simulink model "DroneControlSimulink"  (R2023a)
settings: Solver=ode5  StartTime=0.0  StopTime=30  FixedStep=0.01  RelTol=1e-3
values from neighbouring files (symbols this model uses):
  A = eval(A)    [DroneControlm.m]
  A_o = eval(A_o)    [DroneControlm.m]
  B = eval(B)    [DroneControlm.m]
  B_o = eval(B_o)    [DroneControlm.m]
  C = [1 0 0 0 0 0;0 0 1 0 0 0]    [DroneControlm.m]
  C_o = [1 0 0 0 0 0 0 1 ;0 0 1 0 0 0 1 0]    [DroneControlm.m]
  g = 9.81    [DroneControlm.m]
  h = 0.2    [DroneControlm.m]
  I = 0.003    [DroneControlm.m]
  Ic_xl = [0;0;0;0;0;0]    [DroneControlm.m]
  Ic_xnl = Ic_xl+x_nom    [DroneControlm.m]
  K = lqr(Ab,Bb,Q,R)    [DroneControlm.m]
  L = 0.35    [DroneControlm.m]
  L_o = place(A_o',C_o',D_o)'    [DroneControlm.m]
  m = 1.0    (= 1)    [DroneControlm.m]
  u_nom = eval(u_nom)    [DroneControlm.m]
  x_nom = double(x_nom)    [DroneControlm.m]
libraries: vrlib x2, robotcorelib x1
settings Model: Creator=emuca  LastModifiedBy=omert
settings SolverCC: AlgebraicLoopSolver=TrustRegion
settings DebuggingCC: UnconnectedInputMsg=warning  UnconnectedOutputMsg=warning  UnconnectedLineMsg=warning
settings ModelReferenceCC: EnableRefExpFcnMdlSchedulingChecks=on
settings RTWCC: DLArmComputeVersion=19.05

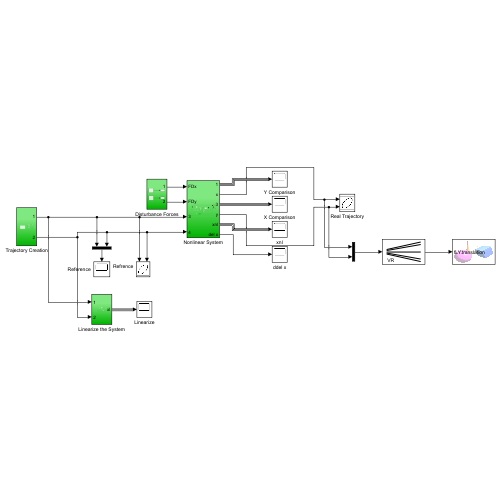
[thumbnail: Simulink's stored preview of the top-level diagram]
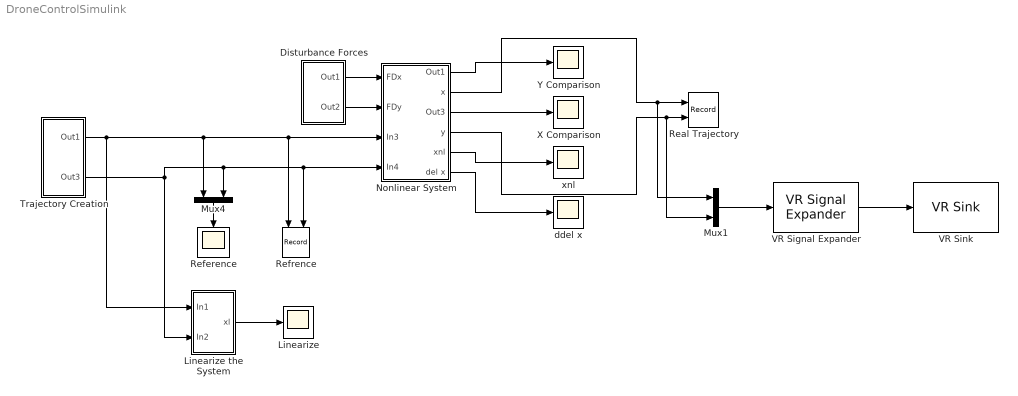
== system DroneControlSimulink ==
  Disturbance Forces : Subsystem
  Linearize : Scope
  Linearize the System : Subsystem
  Mux1 : Mux  Inputs=2
  Mux4 : Mux  Inputs=2
  Nonlinear System : Subsystem
  Real Trajectory : Record  FileSettingsInternal="{\"entries\":[{\"content\":{\"excelSettings\":{\"content\":{},\"type\":\"Streamout.ExcelSettings\"}},\"type\":\"Streamout.FileSettingStorage\",\"uuid\":\"\"}],\"packageUris\":[\"http:\\/\\/schema.mathworks.com\\/mf0\\/streamout_blocks\\/R2020a\"],\"version\":\"1.0\"}"  Layout=[1 1]  SignalsInternal="{\"entries\":[{\"content\":{\"signals\":[{\"content\":{\"blockPath\":[],\"dimensions\":[1],\"domain\":\"\",\"lineColor\":\"#a2142f\",\"plots\":[1],\"port\":1,\"sid\":[\"\"],\"signalID\":4664,\"signalName\":\"Nonlinear System:2\"},\"type\":\"RecordBlkView.Signal\",\"uuid\":\"\"},{\"content\":{\"blockPath\":[],\"dimensions\":[1],\"domain\":\"\",\"lineColor\":\"#139fff\",\"plots\":[1],\"port\":2,\"sid\":[\"\"],\"signalID\":4668,\"signalName\":\"Nonlinear System:4\"},\"type\":\"RecordBlkView.Signal\",\"uuid\":\"\"}]},\"type\":\"RecordBlkView.InputSignals\",\"uuid\":\"\"}],\"packageUris\":[\"http:\\/\\/schema.mathworks.com\\/mf0\\/streamout_blocks\\/R2020a\"],\"version\":\"1.0\"}"  VisualizationBindings="{\"xyplotplugin\":{\"info\":[{\"series\":[{\"bindingParametersList\":[{\"parameter\":\"X-Axis\",\"signalID\":4664,\"signalName\":\"Nonlinear System:2\"},{\"parameter\":\"Y-Axis\",\"signalID\":4668,\"signalName\":\"Nonlinear System:4\"}],\"seriesID\":43140}],\"subplotID\":1}]}}"  CompatibilityTag=XY  st=-1
  Reference : Scope
  "Refrence " : Record  FileSettingsInternal="{\"entries\":[{\"content\":{\"excelSettings\":{\"content\":{},\"type\":\"Streamout.ExcelSettings\"}},\"type\":\"Streamout.FileSettingStorage\",\"uuid\":\"\"}],\"packageUris\":[\"http:\\/\\/schema.mathworks.com\\/mf0\\/streamout_blocks\\/R2020a\"],\"version\":\"1.0\"}"  Layout=[1 1]  SignalsInternal="{\"entries\":[{\"content\":{\"signals\":[{\"content\":{\"blockPath\":[],\"dimensions\":[1],\"domain\":\"\",\"lineColor\":\"#a2142f\",\"plots\":[1],\"port\":1,\"sid\":[\"\"],\"signalID\":4672,\"signalName\":\"Trajectory Creation:1\"},\"type\":\"RecordBlkView.Signal\",\"uuid\":\"\"},{\"content\":{\"blockPath\":[],\"dimensions\":[1],\"domain\":\"\",\"lineColor\":\"#139fff\",\"plots\":[1],\"port\":2,\"sid\":[\"\"],\"signalID\":4676,\"signalName\":\"Trajectory Creation:2\"},\"type\":\"RecordBlkView.Signal\",\"uuid\":\"\"}]},\"type\":\"RecordBlkView.InputSignals\",\"uuid\":\"\"}],\"packageUris\":[\"http:\\/\\/schema.mathworks.com\\/mf0\\/streamout_blocks\\/R2020a\"],\"version\":\"1.0\"}"  VisualizationBindings="{\"xyplotplugin\":{\"info\":[{\"series\":[{\"bindingParametersList\":[{\"parameter\":\"X-Axis\",\"signalID\":4672,\"signalName\":\"Trajectory Creation:1\"},{\"parameter\":\"Y-Axis\",\"signalID\":4676,\"signalName\":\"Trajectory Creation:2\"}],\"seriesID\":33322}],\"subplotID\":1}]}}"  CompatibilityTag=XY  st=-1
  Trajectory Creation : Subsystem
  VR Signal Expander : vrlib/VR Signal Expander  outwidth=3  outidx=[1 2]
  VR Sink : vrlib/VR Sink  InstantiateOnLoad=on  SampleTime=0.1  ViewEnable=on  RemoteChange=off  RemoteView=off  FieldsWritten=fLY.translation.3.1.1.double  WorldFileName=C:\Users\omert\Documents\MATLAB\vrml1.wrl  AutoView=off  VideoDimensions=[]  AllowVariableSize=off
  X Comparison : Scope
  Y Comparison : Scope
  ddel x : Scope
  xnl : Scope
  wires:
  Mux4/1 -> Reference/1
  Trajectory Creation/2(Out3) -> Mux4/2, Nonlinear System/4(In4), "Refrence "/2, Linearize the System/2(In2)
  Trajectory Creation/1(Out1) -> Linearize the System/1(In1), Nonlinear System/3(In3), "Refrence "/1, Mux4/1
  Linearize the System/1(xl) -> Linearize/1
  Disturbance Forces/1(Out1) -> Nonlinear System/1(FDx)
  Disturbance Forces/2(Out2) -> Nonlinear System/2(FDy)
  Nonlinear System/1(Out1) -> Y Comparison/1
  Nonlinear System/2(x) -> Mux1/1, Real Trajectory/1
  Nonlinear System/3(Out3) -> X Comparison/1
  Nonlinear System/4(y) -> Mux1/2, Real Trajectory/2
  Nonlinear System/5(xnl) -> xnl/1
  Nonlinear System/6(del x) -> ddel x/1
  Mux1/1 -> VR Signal Expander/1
  VR Signal Expander/1 -> VR Sink/1

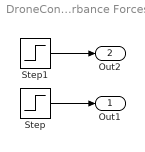
== system DroneControlSimulink/Disturbance Forces ==
  Step : Step  Time=10  SampleTime=0
  Step1 : Step  Time=10  After=0.5  SampleTime=0
  Out1 : Outport
  Out2 : Outport  Port=2
  wires:
  Step/1 -> Out1/1
  Step1/1 -> Out2/1

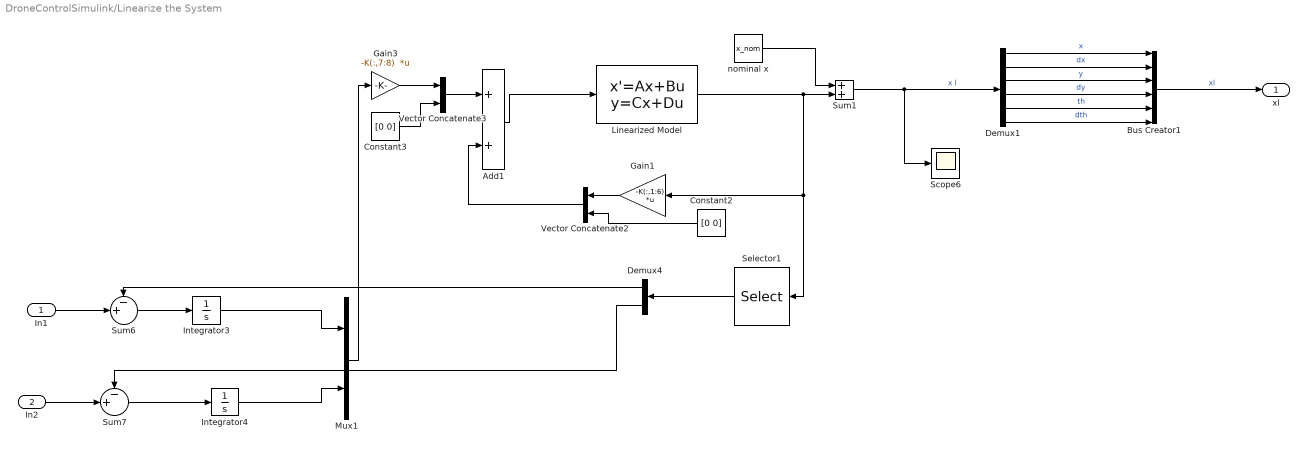
== system DroneControlSimulink/Linearize the System ==
  In1 : Inport
  In2 : Inport  Port=2
  Add1 : Sum  Inputs=2
  Bus Creator1 : BusCreator  Inputs=6
  Constant2 : Constant  Value=[0 0]
  Constant3 : Constant  Value=[0 0]
  Demux1 : Demux  Outputs=6
  Demux4 : Demux  Outputs=2
  Gain1 : Gain  Gain=-K(:,1:6)  Multiplication=Matrix(K*u)
  Gain3 : Gain  Gain=-K(:,7:8)  Multiplication=Matrix(K*u)
  Integrator3 : Integrator
  Integrator4 : Integrator
  Linearized Model : StateSpace  A=A  B=B  C=eye(6)  D=zeros(6,4)  InitialCondition=Ic_xl
  Mux1 : Mux  Inputs=2
  Scope6 : Scope
  Selector1 : Selector  InputPortWidth=6  IndexOptions=Index vector (dialog)  Indices=[1 3]  OutputSizes=1
  Sum1 : Sum
  Sum6 : Sum  Inputs=-+|
  Sum7 : Sum  Inputs=-+|
  Vector Concatenate2 : Concatenate
  Vector Concatenate3 : Concatenate
  nominal x : Constant  Value=x_nom
  xl : Outport
  wires:
  Linearized Model/1 -> Gain1/1, Selector1/1, Sum1/2
  Vector Concatenate2/1 -> Add1/2
  Demux1/6 -> Bus Creator1/6  "dth"
  Sum1/1 -> Scope6/1, Demux1/1  "x l"
  Sum7/1 -> Integrator4/1
  In2/1 -> Sum7/2
  nominal x/1 -> Sum1/1
  Demux1/3 -> Bus Creator1/3  "y"
  Gain1/1 -> Vector Concatenate2/1
  Mux1/1 -> Gain3/1
  Demux4/2 -> Sum7/1
  Integrator4/1 -> Mux1/2
  Demux1/4 -> Bus Creator1/4  "dy"
  Constant3/1 -> Vector Concatenate3/2
  Demux1/5 -> Bus Creator1/5  "th"
  Demux4/1 -> Sum6/1
  Vector Concatenate3/1 -> Add1/1
  Sum6/1 -> Integrator3/1
  Integrator3/1 -> Mux1/1
  In1/1 -> Sum6/2
  Add1/1 -> Linearized Model/1
  Demux1/1 -> Bus Creator1/1  "x"
  Selector1/1 -> Demux4/1
  Demux1/2 -> Bus Creator1/2  "dx"
  Gain3/1 -> Vector Concatenate3/1
  Constant2/1 -> Vector Concatenate2/2
  Bus Creator1/1 -> xl/1  "xl"

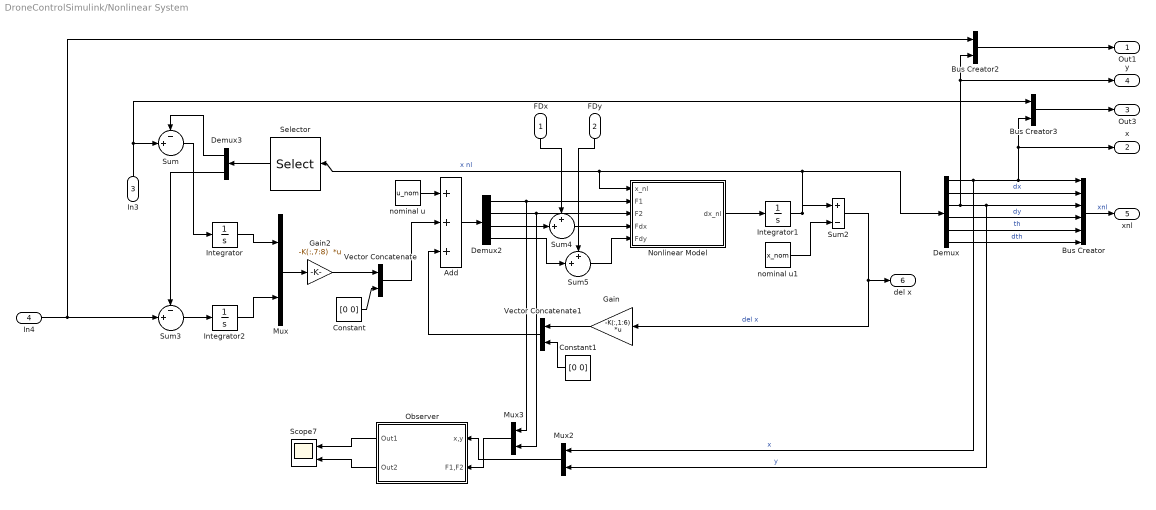
== system DroneControlSimulink/Nonlinear System ==
  FDx : Inport
  FDy : Inport  Port=2
  In3 : Inport  Port=3
  In4 : Inport  Port=4
  Add : Sum  Inputs=3
  Bus Creator : BusCreator  Inputs=6
  Bus Creator2 : BusCreator  Inputs=2
  Bus Creator3 : BusCreator  Inputs=2
  Constant : Constant  Value=[0 0]
  Constant1 : Constant  Value=[0 0]
  Demux : Demux  Outputs=6
  Demux2 : Demux
  Demux3 : Demux  Outputs=2
  Gain : Gain  Gain=-K(:,1:6)  Multiplication=Matrix(K*u)
  Gain2 : Gain  Gain=-K(:,7:8)  Multiplication=Matrix(K*u)
  Integrator : Integrator
  Integrator1 : Integrator  InitialCondition=Ic_xnl
  Integrator2 : Integrator
  Mux : Mux  Inputs=2
  Mux2 : Mux  Inputs=2
  Mux3 : Mux  Inputs=2
  Nonlinear Model : MATLAB Function  TreatAsAtomicUnit=on
  Observer : Subsystem
  Scope7 : Scope  NumInputPorts=2
  Selector : Selector  InputPortWidth=6  IndexOptions=Index vector (dialog)  Indices=[1 3]  OutputSizes=1
  Sum : Sum  Inputs=-+|
  Sum2 : Sum  Inputs=|+-
  Sum3 : Sum  Inputs=-+|
  Sum4 : Sum  Inputs=++|
  Sum5 : Sum  Inputs=++|
  Vector Concatenate : Concatenate
  Vector Concatenate1 : Concatenate
  nominal u : Constant  Value=u_nom
  nominal u1 : Constant  Value=x_nom
  Out1 : Outport
  x : Outport  Port=2
  Out3 : Outport  Port=3
  y : Outport  Port=4
  xnl : Outport  Port=5
  del x : Outport  Port=6
  wires:
  Gain/1 -> Vector Concatenate1/1
  Vector Concatenate/1 -> Add/2
  Nonlinear Model/1(dx_nl) -> Integrator1/1
  In4/1 -> Bus Creator2/1, Sum3/2
  Demux/1 -> x/1, Bus Creator3/2, Bus Creator/1, Mux2/1  "x"
  Sum5/1 -> Nonlinear Model/5(Fdy)
  Sum2/1 -> del x/1, Gain/1  "del x"
  Gain2/1 -> Vector Concatenate/1
  Integrator1/1 -> Selector/1, Nonlinear Model/1(x_nl), Demux/1, Sum2/1  "x nl"
  Demux3/1 -> Sum/1
  Demux2/1 -> Nonlinear Model/2(F1), Mux3/1
  Sum/1 -> Integrator/1
  FDx/1 -> Sum4/1
  nominal u/1 -> Add/1
  Mux3/1 -> Observer/2(F1,F2)
  nominal u1/1 -> Sum2/2
  Vector Concatenate1/1 -> Add/3
  Integrator2/1 -> Mux/2
  Demux3/2 -> Sum3/1
  Demux2/4 -> Sum5/2
  Mux/1 -> Gain2/1
  Constant1/1 -> Vector Concatenate1/2
  Integrator/1 -> Mux/1
  Add/1 -> Demux2/1
  Observer/1(Out1) -> Scope7/1
  Demux/2 -> Bus Creator/2  "dx"
  Mux2/1 -> Observer/1(x,y)
  Bus Creator2/1 -> Out1/1
  Demux2/2 -> Mux3/2, Nonlinear Model/3(F2)
  Sum4/1 -> Nonlinear Model/4(Fdx)
  Demux/3 -> Bus Creator/3, Mux2/2, Bus Creator2/2, y/1  "y"
  Demux/5 -> Bus Creator/5  "th"
  Observer/2(Out2) -> Scope7/2
  In3/1 -> Sum/2, Bus Creator3/1
  Demux2/3 -> Sum4/2
  Constant/1 -> Vector Concatenate/2
  Bus Creator/1 -> xnl/1  "xnl"
  Selector/1 -> Demux3/1
  Sum3/1 -> Integrator2/1
  Demux/6 -> Bus Creator/6  "dth"
  Demux/4 -> Bus Creator/4  "dy"
  Bus Creator3/1 -> Out3/1
  FDy/1 -> Sum5/1

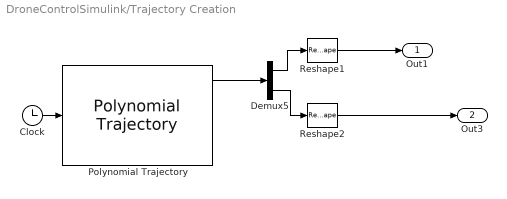
== system DroneControlSimulink/Trajectory Creation ==
  Clock : Clock
  Demux5 : Demux  Outputs=2
  Polynomial Trajectory : robotcorelib/Polynomial Trajectory  WaypointSource=Internal  Waypoints=[0,0,0,0,0,2,4,6,8,10,10,10,10,10,12,13.5,13.5,13.5,13.5,13.5,14.5,15.5,15.5;0,1,2,3,4,4,4,4,4,4,3,2,1,0,0,0,1,2,3,4,4,4,3]  TimePoints=[0,1,2,3,4,5,6,7,8,9,10,11,12,13,14,15,16,17,18,19,20,21,22]  TimeInterval=[ 1, 4 ]  Method=Cubic Polynomial  ParameterSource=Internal  VelocityBoundaryCondition=zeros( 2, 23 )  AccelerationBoundaryCondition=zeros( 2, 7 )  SimulateUsing=Interpreted execution
  Reshape1 : Reshape
  Reshape2 : Reshape
  Out1 : Outport
  Out3 : Outport  Port=2
  wires:
  Demux5/2 -> Reshape2/1
  Demux5/1 -> Reshape1/1
  Clock/1 -> Polynomial Trajectory/1
  Reshape1/1 -> Out1/1
  Polynomial Trajectory/1 -> Demux5/1
  Reshape2/1 -> Out3/1

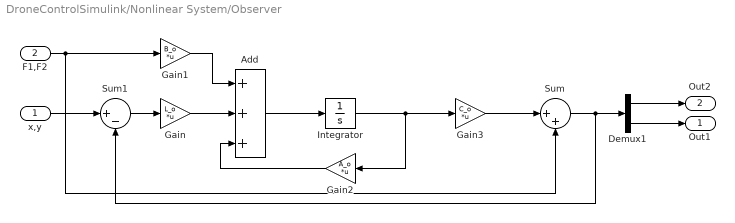
== system DroneControlSimulink/Nonlinear System/Observer ==
  x,y : Inport
  F1,F2 : Inport  Port=2
  Add : Sum  Inputs=3
  Demux1 : Demux  Outputs=2
  Gain : Gain  Gain=L_o  Multiplication=Matrix(K*u)
  Gain1 : Gain  Gain=B_o  Multiplication=Matrix(K*u)
  Gain2 : Gain  Gain=A_o  Multiplication=Matrix(K*u)
  Gain3 : Gain  Gain=C_o  Multiplication=Matrix(K*u)
  Integrator : Integrator
  Sum : Sum  Inputs=|++
  Sum1 : Sum  Inputs=|+-
  Out1 : Outport
  Out2 : Outport  Port=2
  wires:
  x,y/1 -> Sum1/1
  Sum1/1 -> Gain/1
  Gain/1 -> Add/2
  F1,F2/1 -> Sum/2, Gain1/1
  Gain1/1 -> Add/1
  Add/1 -> Integrator/1
  Integrator/1 -> Gain3/1, Gain2/1
  Gain2/1 -> Add/3
  Gain3/1 -> Sum/1
  Sum/1 -> Demux1/1, Sum1/2
  Demux1/1 -> Out2/1
  Demux1/2 -> Out1/1

== matlab function DroneControlSimulink/Nonlinear System/Nonlinear Model ==
  data: x_nl input; h parameter; L parameter; g parameter; I parameter; dx_nl output; m parameter; F1 input; F2 input; Fdx input; Fdy input
function dx_nl = fcn(x_nl,h, L, g, I, m, F1, F2,Fdx,Fdy)

x=x_nl(1);
dx=x_nl(2);
y=x_nl(3);
dy=x_nl(4);
th=x_nl(5);
dth=x_nl(6);



f_ddx= (-(F1+F2)*sin(th)+Fdx)/m;
f_ddy= ((F1+F2)*cos(th)-m*g+Fdy)/m;
f_ddth=((F1-F2)*L+Fdx*h*cos(th)+Fdy*h*sin(th))/I;


dx_nl=[dx;f_ddx;dy;f_ddy;dth;f_ddth];
